simulink model "bdcMotor_control"  (R2018a)
settings: Solver=VariableStepAuto  StartTime=0.0  StopTime=0.1  RelTol=1e-3
model workspace (MAT data in the model file):
  Bm = 3.1346e-05
  Jm = 6.88627e-06
  Kb = 0.0583
  Ki = 0.0583
  La = 0.003694
  Ra = 5.385
settings Model: Creator=Kim  LastModifiedBy=Kim

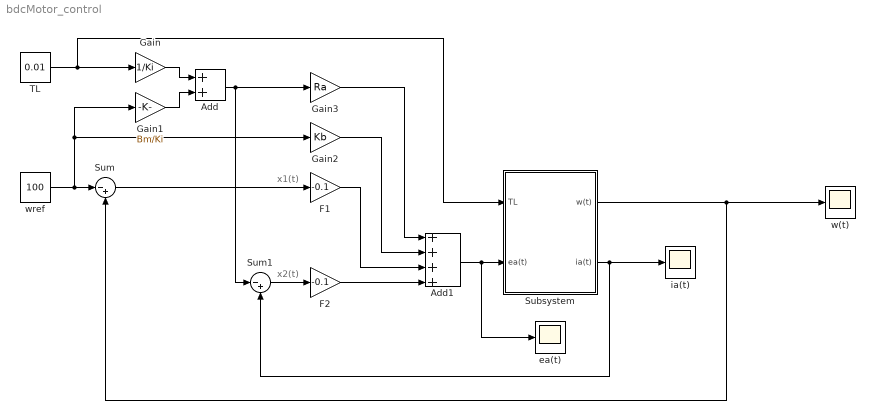
== system bdcMotor_control ==
  note: x1(t)
  note: x2(t)
  Add : Sum
  Add1 : Sum  Inputs=++++
  F1 : Gain  Gain=-0.1
  F2 : Gain  Gain=-0.1
  Gain : Gain  Gain=1/Ki
  Gain1 : Gain  Gain=Bm/Ki
  Gain2 : Gain  Gain=Kb
  Gain3 : Gain  Gain=Ra
  Subsystem : Subsystem
  Sum : Sum  Inputs=|-+
  Sum1 : Sum  Inputs=|-+
  TL : Constant  Value=0.01
  ea(t) : Scope
  ia(t) : Scope
  w(t) : Scope
  wref : Constant  Value=100
  wires:
  wref/1 -> Gain2/1, Gain1/1, Sum/1
  Subsystem/1(w(t)) -> w(t)/1, Sum/2
  Gain/1 -> Add/1
  Gain1/1 -> Add/2
  Add/1 -> Gain3/1, Sum1/1
  Subsystem/2(ia(t)) -> ia(t)/1, Sum1/2
  Sum/1 -> F1/1
  Sum1/1 -> F2/1
  F2/1 -> Add1/4
  F1/1 -> Add1/3
  Gain3/1 -> Add1/1
  Gain2/1 -> Add1/2
  Add1/1 -> ea(t)/1, Subsystem/2(ea(t))
  TL/1 -> Subsystem/1(TL), Gain/1

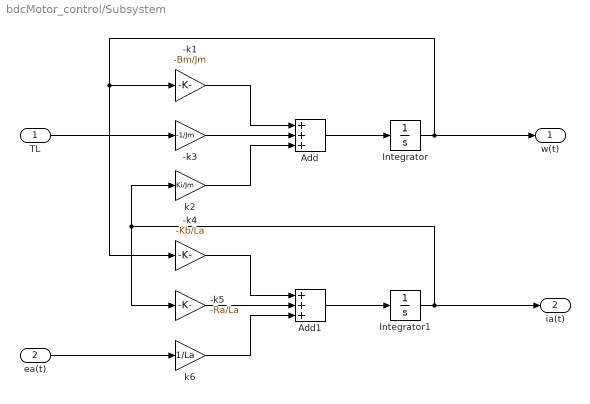
== system bdcMotor_control/Subsystem ==
  TL : Inport
  ea(t) : Inport  Port=2
  -k1 : Gain  Gain=-Bm/Jm
  -k3 : Gain  Gain=-1/Jm
  -k4 : Gain  Gain=-Kb/La
  -k5 : Gain  Gain=-Ra/La
  Add : Sum  Inputs=+++
  Add1 : Sum  Inputs=+++
  Integrator : Integrator
  Integrator1 : Integrator
  k2 : Gain  Gain=Ki/Jm
  k6 : Gain  Gain=1/La
  w(t) : Outport
  ia(t) : Outport  Port=2
  wires:
  -k5/1 -> Add1/2
  -k4/1 -> Add1/1
  -k1/1 -> Add/1
  k6/1 -> Add1/3
  -k3/1 -> Add/2
  Add/1 -> Integrator/1
  Integrator/1 -> w(t)/1, -k4/1, -k1/1
  Add1/1 -> Integrator1/1
  Integrator1/1 -> ia(t)/1, -k5/1, k2/1
  ea(t)/1 -> k6/1
  k2/1 -> Add/3
  TL/1 -> -k3/1
